simulink model "Pub_Sub_Husqvarna_Const"  (R2017a)
settings: Solver=VariableStepAuto  StartTime=0.0  StopTime=inf  RelTol=1e-3
undefined symbols (not defined in the file): Angular, Linear
libraries: robotlib x2, fuzblock x1
settings Model: Creator=francesco  LastModifiedBy=francesco

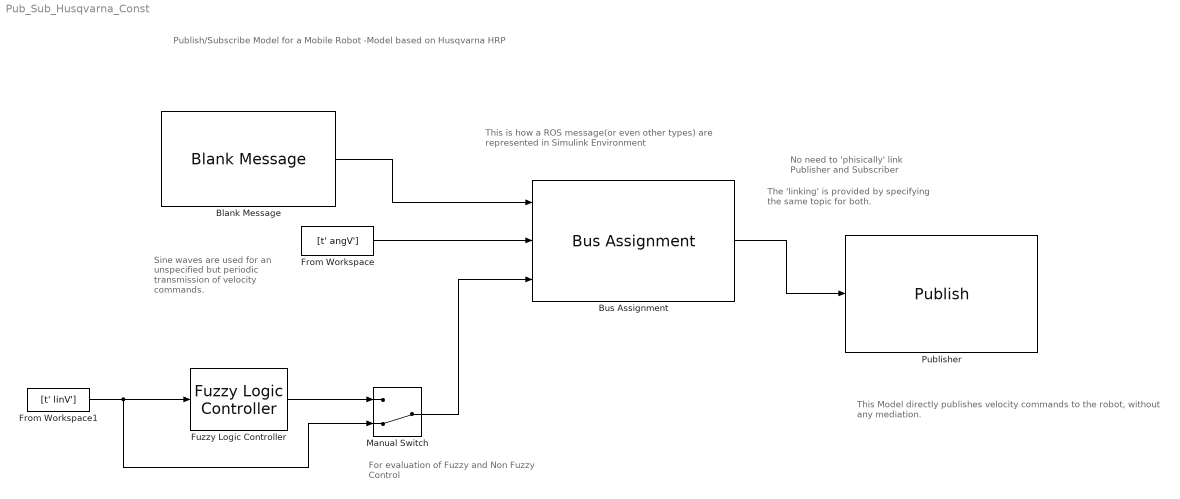
== system Pub_Sub_Husqvarna_Const ==
  note: This Model directly publishes velocity commands to the
      | robot, without any mediation.
  note: Publish/Subscribe Model for a Mobile Robot
      | -Model based on Husqvarna HRP
  note: Sine waves are used for an
      | unspecified but periodic
      | transmission of velocity
      | commands.
  note: No need to 'phisically' link
      | Publisher and Subscriber
  note: The 'linking' is provided by specifying
      | the same topic for both.
  note: This is how a ROS message(or even other types)
      |  are represented in Simulink Environment
  note: For evaluation of Fuzzy and Non Fuzzy
      | Control
  Blank Message : robotlib/Blank Message  SourceLibraryInfo=This block requires Robotics System Toolbox  messageType=geometry_msgs/Twist  SampleTime=inf
      settings: SourceProductBaseCode=RO
  Bus Assignment : BusAssignment  AssignedSignals=Linear.X,Angular.Z
  From Workspace : FromWorkspace  VariableName=[t' angV']  OutDataTypeStr=double  SampleTime=0  Interpolate=off  OutputAfterFinalValue=Setting to zero
  From Workspace1 : FromWorkspace  VariableName=[t' linV']  OutDataTypeStr=double  SampleTime=0  Interpolate=off  OutputAfterFinalValue=Setting to zero
  Fuzzy Logic Controller : fuzblock/Fuzzy Logic  Controller  fis='LinVelDefinitivo.fis'
  Manual Switch : ManualSwitch  CurrentSetting=0
  Publisher : robotlib/Publish  SourceLibraryInfo=This block requires Robotics System Toolbox  topicSource=Select from ROS network  topic=/cmd_vel  messageType=geometry_msgs/Twist  messageQueueLength=1
      settings: SourceProductBaseCode=RO
  wires:
  Manual Switch/1 -> Bus Assignment/3
  Blank Message/1 -> Bus Assignment/1
  From Workspace/1 -> Bus Assignment/2
  Fuzzy Logic Controller/1 -> Manual Switch/1
  From Workspace1/1 -> Manual Switch/2, Fuzzy Logic Controller/1
  Bus Assignment/1 -> Publisher/1
